simulink subsystem "DronePlantSubsystem"  (R2023b)
settings: Solver=VariableStepAuto  StartTime=0.0  StopTime=10.0  RelTol=1e-3
values from neighbouring files (symbols this model uses):
  Ax = 0.0    (= 0)    [drone_input_params.m]
  Ay = 0.0    (= 0)    [drone_input_params.m]
  Az = 0.0    (= 0)    [drone_input_params.m]
  b = 192.3208*10^(-7)    (= 1.923208e-05)    [drone_input_params.m]
  d = 4.003*10^(-7)    (= 4.003e-07)    [drone_input_params.m]
  g = 9.81    [drone_input_params.m]
  Ixx = 15.67*10^(-3)    (= 0.01567)    [drone_input_params.m]
  Iyy = 15.67*10^(-3)    (= 0.01567)    [drone_input_params.m]
  Izz = 28.346*10^(-3)    (= 0.028346)    [drone_input_params.m]
  Jr = 6.01*10^(-5)    (= 6.01e-05)    [drone_input_params.m]
  l = 0.3    [drone_input_params.m]
  m = weight/g    (= 0.815494393476)    [drone_input_params.m]
settings Model: Creator=FRESH  LastModifiedBy=FRESH

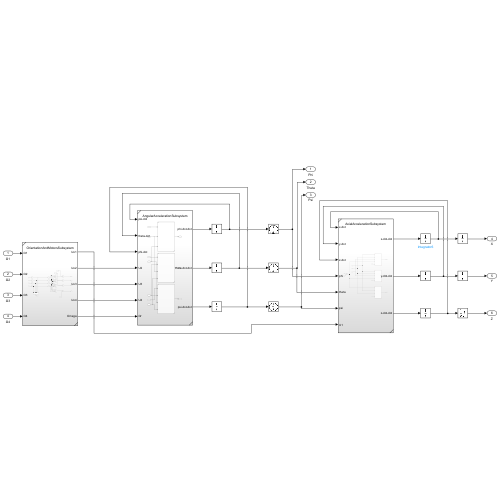
[thumbnail: Simulink's stored preview of the top-level diagram]
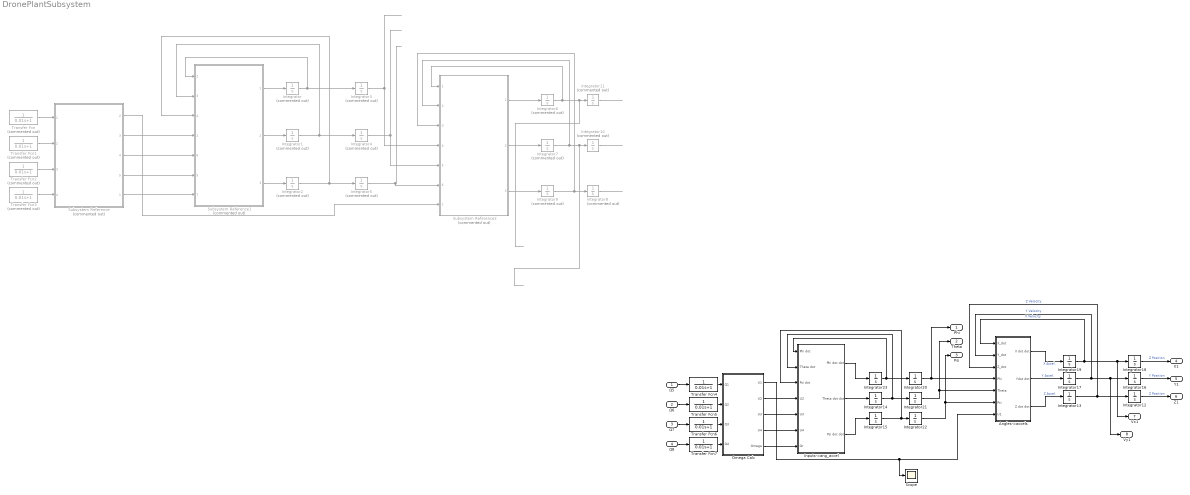
== system DronePlantSubsystem ==
  Ω5 : Inport
  Ω6 : Inport  Port=2
  Ω7 : Inport  Port=3
  Ω8 : Inport  Port=4
  Angles->accels : Subsystem
  Inputs->ang_accel : Subsystem
  Integrator{,1..2,6..7,9..11} (8 alike) : Integrator  Commented=on
  Integrator12 : Integrator  LimitOutput=on  LowerSaturationLimit=0
  Integrator{13,16..19,22..23} (7 alike) : Integrator
  Integrator14 : Integrator  UpperSaturationLimit=10000  LowerSaturationLimit=-10000
  Integrator15 : Integrator  UpperSaturationLimit=10000  LowerSaturationLimit=-10000
  Integrator20 : Integrator  WrapState=on  WrappedStateUpperValue=pi/2  WrappedStateLowerValue=-pi/2
  Integrator21 : Integrator  WrapState=on  WrappedStateUpperValue=pi/3  WrappedStateLowerValue=-pi/3
  Integrator3 : Integrator  Commented=on  WrapState=on
  Integrator4 : Integrator  Commented=on  WrapState=on
  Integrator5 : Integrator  Commented=on  WrapState=on
  Integrator8 : Integrator  Commented=on  LimitOutput=on  UpperSaturationLimit=0
  Omega Calc : Subsystem
  Scope : Scope
  Subsystem Reference : Subsystem  Commented=on  ReferencedSubsystem=OrientationAndMotorsSubsystem
      settings: PortSchema="{\"entries\":[{\"content\":{\"sides\":[{\"content\":{\"connectorIds\":[\"In1\",\"In2\",\"In3\",\"In4\"]},\"type\":\"ConnectorPlacement.EquallySpacedRectSide\",\"uuid\":\"54093c14-6905-4315-89a2-d57263587d77\"},{\"content\":{\"connectorIds\":[\"Out2\",\"Out3\",\"Out4\",\"Out5\",\"Out1\"],\"side\":\"RIGHT\"},\"type\":\"ConnectorPlacement.EquallySpacedRectSide\",\"uuid\":\"792b5cf1-0f94-4e71-8b93-1e59081231d9\"},{\"content\":{\"side\":\"TOP\"},\"type\":\"ConnectorPlacement.EquallySpacedRectSide\",\"uuid\":\"8a70e999-dff0-4dcb-8d8e-633240736e28\"}]},\"type\":\"ConnectorPlacement.EquallySpacedConnector\",\"uuid\":\"4c2f7de4-146f-41b0-aabc-cf54c6108d54\"}],\"packageUris\":[\"http://schema.mathworks.com/mf0/Connector/R2020b\"],\"version\":\"1.0\"}"
  Subsystem Reference1 : Subsystem  Commented=on  ReferencedSubsystem=AngularAccelerationSubsystem
      settings: PortSchema="{\"entries\":[{\"content\":{\"sides\":[{\"content\":{\"connectorIds\":[\"In2\",\"In3\",\"In4\",\"In1\",\"In6\",\"In5\",\"In7\"]},\"type\":\"ConnectorPlacement.EquallySpacedRectSide\",\"uuid\":\"e7cd80e4-513a-49bb-8a32-93ee463d1d18\"},{\"content\":{\"connectorIds\":[\"Out1\",\"Out2\",\"Out3\"],\"side\":\"RIGHT\"},\"type\":\"ConnectorPlacement.EquallySpacedRectSide\",\"uuid\":\"416d32a0-b191-4ff2-830a-04dcaeaab673\"},{\"content\":{\"side\":\"TOP\"},\"type\":\"ConnectorPlacement.EquallySpacedRectSide\",\"uuid\":\"e39a2d85-751d-4d15-b0f4-13a7a5828542\"}]},\"type\":\"ConnectorPlacement.EquallySpacedConnector\",\"uuid\":\"cd683958-b96b-4e10-be5c-088f75616717\"}],\"packageUris\":[\"http://schema.mathworks.com/mf0/Connector/R2020b\"],\"version\":\"1.0\"}"
  Subsystem Reference2 : Subsystem  Commented=on  ReferencedSubsystem=AxialAccelerationSubsystem
  Transfer Fcn{,1..3} (4 alike) : TransferFcn  Commented=on  Denominator=[0.01 1]
  Transfer Fcn{4..7} (4 alike) : TransferFcn  Denominator=[0.01 1]
  Phi : Outport  VectorParamsAs1DForOutWhenUnconnected=off
  Theta : Outport  Port=2  VectorParamsAs1DForOutWhenUnconnected=off
  Psi : Outport  Port=3  VectorParamsAs1DForOutWhenUnconnected=off
  X1 : Outport  Port=4  VectorParamsAs1DForOutWhenUnconnected=off
  Y1 : Outport  Port=5  VectorParamsAs1DForOutWhenUnconnected=off
  Z1 : Outport  Port=6  VectorParamsAs1DForOutWhenUnconnected=off
  Vx1 : Outport  Port=7  VectorParamsAs1DForOutWhenUnconnected=off
  Vy1 : Outport  Port=8  VectorParamsAs1DForOutWhenUnconnected=off
  wires:
  ? -> Transfer Fcn/1
  ? -> Transfer Fcn1/1
  ? -> Transfer Fcn2/1
  ? -> Transfer Fcn3/1
  Subsystem Reference/1 -> Subsystem Reference1/7
  Subsystem Reference/5 -> Subsystem Reference1/5
  Subsystem Reference/4 -> Subsystem Reference1/6
  Subsystem Reference/3 -> Subsystem Reference1/1
  Subsystem Reference1/1 -> Integrator/1
  Subsystem Reference1/2 -> Integrator1/1
  Subsystem Reference1/3 -> Integrator2/1
  Integrator/1 -> Integrator3/1, Subsystem Reference1/2
  Integrator1/1 -> Subsystem Reference1/3, Integrator4/1
  Integrator2/1 -> Subsystem Reference1/4, Integrator5/1
  Integrator5/1 -> Subsystem Reference2/6
  Integrator4/1 -> Subsystem Reference2/5
  Integrator3/1 -> Subsystem Reference2/4
  Subsystem Reference/2 -> Subsystem Reference2/7
  Subsystem Reference2/1 -> Integrator6/1
  Subsystem Reference2/2 -> Integrator7/1
  Subsystem Reference2/3 -> Integrator9/1
  Integrator7/1 -> Subsystem Reference2/2, Integrator10/1
  Integrator9/1 -> Integrator8/1, Subsystem Reference2/3
  Integrator11/1 -> ?
  Integrator10/1 -> ?
  Integrator8/1 -> ?
  Integrator6/1 -> Integrator11/1, Subsystem Reference2/1
  Transfer Fcn/1 -> Subsystem Reference/1
  Transfer Fcn1/1 -> Subsystem Reference/2
  Transfer Fcn2/1 -> Subsystem Reference/3
  Transfer Fcn3/1 -> Subsystem Reference/4
  Omega Calc/4(U4) -> Inputs->ang_accel/6(U4)
  Angles->accels/1(X dot dot) -> Integrator19/1  "X Accel."
  Ω8/1 -> Transfer Fcn7/1
  Ω7/1 -> Transfer Fcn6/1
  Transfer Fcn4/1 -> Omega Calc/1(Ω1)
  Omega Calc/5(Omega) -> Inputs->ang_accel/7(Ωr)
  Integrator18/1 -> X1/1  "Z Position"
  Ω5/1 -> Transfer Fcn4/1
  Integrator15/1 -> Integrator22/1, Inputs->ang_accel/3(Psi dot)
  Ω6/1 -> Transfer Fcn5/1
  Transfer Fcn5/1 -> Omega Calc/2(Ω2)
  Integrator23/1 -> Integrator20/1, Inputs->ang_accel/1(Phi dot)
  Integrator19/1 -> Integrator18/1, Vx1/1, Angles->accels/1(X_dot)  "X Velocity"
  Integrator20/1 -> Phi/1, Angles->accels/4(Phi)
  Inputs->ang_accel/3(Psi dot dot) -> Integrator15/1
  Inputs->ang_accel/1(Phi dot dot) -> Integrator23/1
  Integrator12/1 -> Z1/1  "Z Position"
  Omega Calc/2(U2) -> Inputs->ang_accel/4(U2)
  Integrator14/1 -> Integrator21/1, Inputs->ang_accel/2(Theta dot)
  Angles->accels/3(Z dot dot) -> Integrator13/1  "Z Accel."
  Integrator16/1 -> Y1/1  "Y Position"
  Angles->accels/2(Ydot dot) -> Integrator17/1  "Y Accel."
  Omega Calc/1(U1) -> Angles->accels/7(U1), Scope/1
  Inputs->ang_accel/2(Theta dot dot) -> Integrator14/1
  Transfer Fcn7/1 -> Omega Calc/4(Ω4)
  Integrator17/1 -> Integrator16/1, Vy1/1, Angles->accels/2(Y_dot)  "Y Velocity"
  Integrator13/1 -> Integrator12/1, Angles->accels/3(Z_dot)  "Z Velocity"
  Integrator22/1 -> Psi/1, Angles->accels/6(Psi)
  Transfer Fcn6/1 -> Omega Calc/3(Ω3)
  Integrator21/1 -> Theta/1, Angles->accels/5(Theta)
  Omega Calc/3(U3) -> Inputs->ang_accel/5(U3)

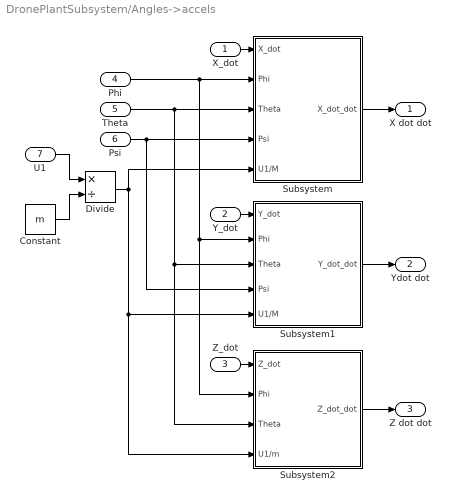
== system DronePlantSubsystem/Angles->accels ==
  X_dot : Inport
  Y_dot : Inport  Port=2
  Z_dot : Inport  Port=3
  Phi : Inport  Port=4
  Theta : Inport  Port=5
  Psi : Inport  Port=6
  U1 : Inport  Port=7
  Constant : Constant  Value=m
  Divide : Product  Inputs=*/
  Subsystem : Subsystem
  Subsystem1 : Subsystem
  Subsystem2 : Subsystem
  X dot dot : Outport  VectorParamsAs1DForOutWhenUnconnected=off
  Ydot dot : Outport  Port=2  VectorParamsAs1DForOutWhenUnconnected=off
  Z dot dot : Outport  Port=3  VectorParamsAs1DForOutWhenUnconnected=off
  wires:
  Z_dot/1 -> Subsystem2/1(Z_dot)
  Y_dot/1 -> Subsystem1/1(Y_dot)
  X_dot/1 -> Subsystem/1(X_dot)
  Psi/1 -> Subsystem/4(Psi), Subsystem1/4(Psi)
  Theta/1 -> Subsystem/3(Theta), Subsystem1/3(Theta), Subsystem2/3(Theta)
  Subsystem2/1(Z_dot_dot) -> Z dot dot/1
  Subsystem1/1(Y_dot_dot) -> Ydot dot/1
  Subsystem/1(X_dot_dot) -> X dot dot/1
  Divide/1 -> Subsystem1/5(U1/M), Subsystem2/4(U1/m), Subsystem/5(U1/M)
  Constant/1 -> Divide/2
  U1/1 -> Divide/1
  Phi/1 -> Subsystem/2(Phi), Subsystem1/2(Phi), Subsystem2/2(Phi)

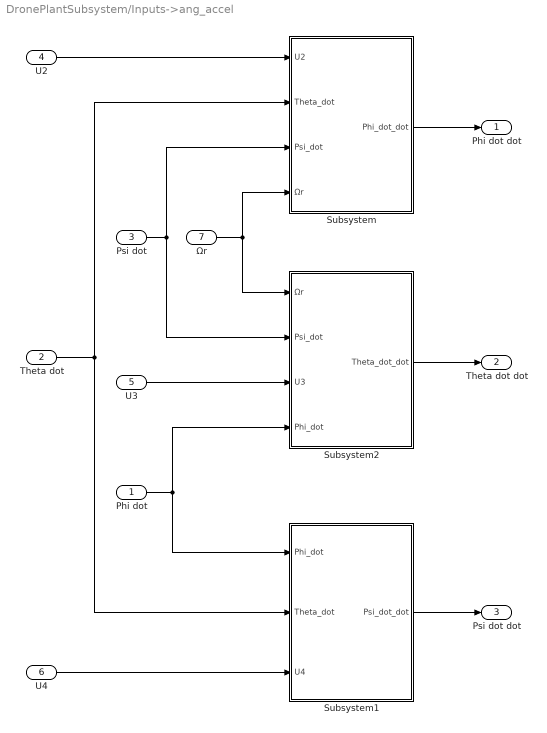
== system DronePlantSubsystem/Inputs->ang_accel ==
  Phi dot : Inport
  Theta dot : Inport  Port=2
  Psi dot : Inport  Port=3
  U2 : Inport  Port=4
  U3 : Inport  Port=5
  U4 : Inport  Port=6
  Ωr : Inport  Port=7
  Subsystem : Subsystem
  Subsystem1 : Subsystem
  Subsystem2 : Subsystem
  Phi dot dot : Outport  VectorParamsAs1DForOutWhenUnconnected=off
  Theta dot dot : Outport  Port=2  VectorParamsAs1DForOutWhenUnconnected=off
  Psi dot dot : Outport  Port=3  VectorParamsAs1DForOutWhenUnconnected=off
  wires:
  Phi dot/1 -> Subsystem1/1(Phi_dot), Subsystem2/4(Phi_dot)
  Theta dot/1 -> Subsystem1/2(Theta_dot), Subsystem/2(Theta_dot)
  Subsystem1/1(Psi_dot_dot) -> Psi dot dot/1
  Subsystem2/1(Theta_dot_dot) -> Theta dot dot/1
  Psi dot/1 -> Subsystem/3(Psi_dot), Subsystem2/2(Psi_dot)
  Ωr/1 -> Subsystem2/1(Ωr), Subsystem/4(Ωr)
  U2/1 -> Subsystem/1(U2)
  Subsystem/1(Phi_dot_dot) -> Phi dot dot/1
  U4/1 -> Subsystem1/3(U4)
  U3/1 -> Subsystem2/3(U3)

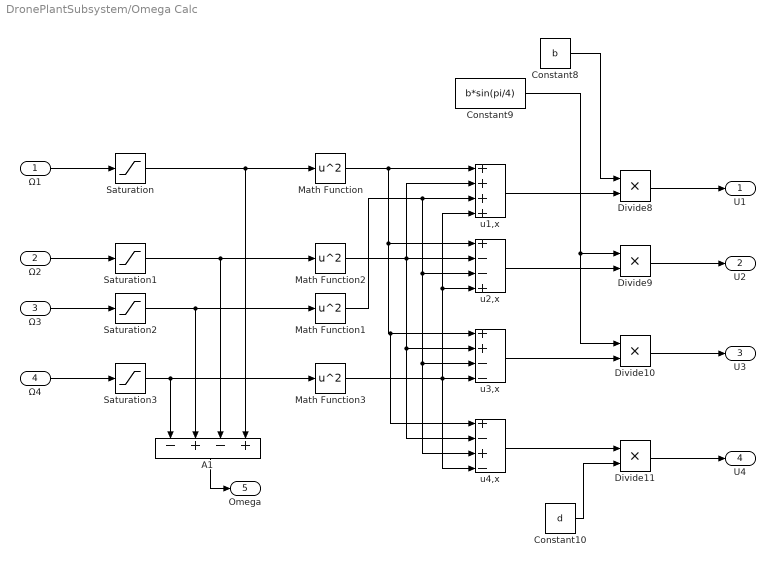
== system DronePlantSubsystem/Omega Calc ==
  Ω1 : Inport
  Ω2 : Inport  Port=2
  Ω3 : Inport  Port=3
  Ω4 : Inport  Port=4
  A1 : Sum  Inputs=-+-+
  Constant10 : Constant  Value=d
  Constant8 : Constant  Value=b
  Constant9 : Constant  Value=b*sin(pi/4)
  Divide{8..11} (4 alike) : Product  Inputs=**
  Math Function{,1..3} (4 alike) : Math  Operator=square  SignedPower=on
  Saturation{,1..3} (4 alike) : Saturate  UpperLimit=inf  LowerLimit=0
  u1,x : Sum  Inputs=++++
  u2,x : Sum  Inputs=+--+
  u3,x : Sum  Inputs=++--
  u4,x : Sum  Inputs=+-+-
  U1 : Outport  VectorParamsAs1DForOutWhenUnconnected=off
  U2 : Outport  Port=2  VectorParamsAs1DForOutWhenUnconnected=off
  U3 : Outport  Port=3  VectorParamsAs1DForOutWhenUnconnected=off
  U4 : Outport  Port=4  VectorParamsAs1DForOutWhenUnconnected=off
  Omega : Outport  Port=5  VectorParamsAs1DForOutWhenUnconnected=off
  wires:
  Saturation3/1 -> Math Function3/1, A1/1
  Saturation/1 -> A1/4, Math Function/1
  Saturation1/1 -> A1/3, Math Function2/1
  Saturation2/1 -> Math Function1/1, A1/2
  Ω4/1 -> Saturation3/1
  Ω3/1 -> Saturation2/1
  Ω2/1 -> Saturation1/1
  Ω1/1 -> Saturation/1
  Math Function3/1 -> u3,x/4, u4,x/4, u2,x/4, u1,x/4
  Math Function2/1 -> u2,x/2, u3,x/2, u4,x/2, u1,x/2
  Math Function1/1 -> u1,x/3, u2,x/3, u3,x/3, u4,x/3
  Math Function/1 -> u1,x/1, u2,x/1, u3,x/1, u4,x/1
  Divide11/1 -> U4/1
  Divide10/1 -> U3/1
  Divide9/1 -> U2/1
  Divide8/1 -> U1/1
  A1/1 -> Omega/1
  Constant8/1 -> Divide8/1
  u1,x/1 -> Divide8/2
  Constant9/1 -> Divide9/1, Divide10/1
  u2,x/1 -> Divide9/2
  u3,x/1 -> Divide10/2
  u4,x/1 -> Divide11/1
  Constant10/1 -> Divide11/2

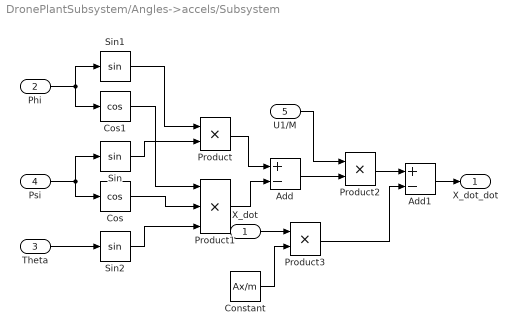
== system DronePlantSubsystem/Angles->accels/Subsystem ==
  X_dot : Inport
  Phi : Inport  Port=2
  Theta : Inport  Port=3
  Psi : Inport  Port=4
  U1/M : Inport  Port=5
  Add : Sum  Inputs=+-
  Add1 : Sum  Inputs=+-
  Constant : Constant  Value=Ax/m
  Cos : Trigonometry  Operator=cos
  Cos1 : Trigonometry  Operator=cos
  Product : Product
  Product1 : Product  Inputs=3
  Product2 : Product
  Product3 : Product
  Sin : Trigonometry
  Sin1 : Trigonometry
  Sin2 : Trigonometry
  X_dot_dot : Outport  VectorParamsAs1DForOutWhenUnconnected=off
  wires:
  Product3/1 -> Add1/2
  Constant/1 -> Product3/2
  X_dot/1 -> Product3/1
  Add1/1 -> X_dot_dot/1
  Product2/1 -> Add1/1
  Sin/1 -> Product/2
  Sin1/1 -> Product/1
  Sin2/1 -> Product1/3
  Cos/1 -> Product1/2
  Cos1/1 -> Product1/1
  Theta/1 -> Sin2/1
  Phi/1 -> Sin1/1, Cos1/1
  Psi/1 -> Sin/1, Cos/1
  Add/1 -> Product2/2
  U1/M/1 -> Product2/1
  Product/1 -> Add/1
  Product1/1 -> Add/2

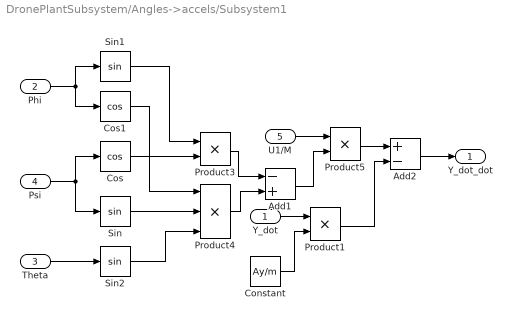
== system DronePlantSubsystem/Angles->accels/Subsystem1 ==
  Y_dot : Inport
  Phi : Inport  Port=2
  Theta : Inport  Port=3
  Psi : Inport  Port=4
  U1/M : Inport  Port=5
  Add1 : Sum  Inputs=-+
  Add2 : Sum  Inputs=+-
  Constant : Constant  Value=Ay/m
  Cos : Trigonometry  Operator=cos
  Cos1 : Trigonometry  Operator=cos
  Product1 : Product
  Product3 : Product
  Product4 : Product  Inputs=3
  Product5 : Product
  Sin : Trigonometry
  Sin1 : Trigonometry
  Sin2 : Trigonometry
  Y_dot_dot : Outport  VectorParamsAs1DForOutWhenUnconnected=off
  wires:
  Add2/1 -> Y_dot_dot/1
  Product5/1 -> Add2/1
  Product1/1 -> Add2/2
  Constant/1 -> Product1/2
  Y_dot/1 -> Product1/1
  Cos/1 -> Product3/2
  Sin1/1 -> Product3/1
  Sin2/1 -> Product4/3
  Sin/1 -> Product4/2
  Cos1/1 -> Product4/1
  Product3/1 -> Add1/1
  U1/M/1 -> Product5/1
  Product4/1 -> Add1/2
  Add1/1 -> Product5/2
  Theta/1 -> Sin2/1
  Phi/1 -> Sin1/1, Cos1/1
  Psi/1 -> Cos/1, Sin/1

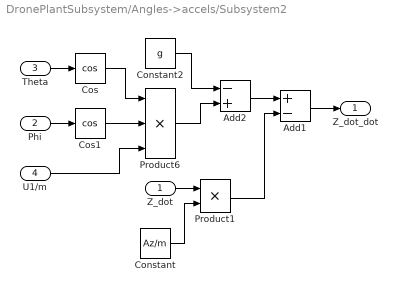
== system DronePlantSubsystem/Angles->accels/Subsystem2 ==
  Z_dot : Inport
  Phi : Inport  Port=2
  Theta : Inport  Port=3
  U1/m : Inport  Port=4
  Add1 : Sum  Inputs=+-
  Add2 : Sum  Inputs=-+
  Constant : Constant  Value=Az/m
  Constant2 : Constant  Value=g
  Cos : Trigonometry  Operator=cos
  Cos1 : Trigonometry  Operator=cos
  Product1 : Product
  Product6 : Product  Inputs=3
  Z_dot_dot : Outport  VectorParamsAs1DForOutWhenUnconnected=off
  wires:
  Add1/1 -> Z_dot_dot/1
  Add2/1 -> Add1/1
  Constant/1 -> Product1/2
  Z_dot/1 -> Product1/1
  Product1/1 -> Add1/2
  Cos1/1 -> Product6/2
  Product6/1 -> Add2/2
  Cos/1 -> Product6/1
  Constant2/1 -> Add2/1
  U1/m/1 -> Product6/3
  Theta/1 -> Cos/1
  Phi/1 -> Cos1/1

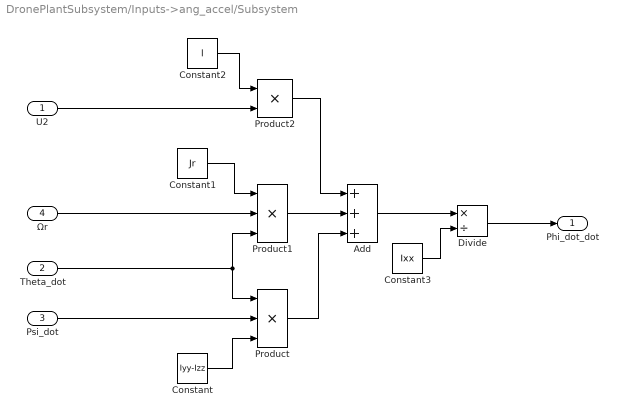
== system DronePlantSubsystem/Inputs->ang_accel/Subsystem ==
  U2 : Inport
  Theta_dot : Inport  Port=2
  Psi_dot : Inport  Port=3
  Ωr : Inport  Port=4
  Add : Sum  Inputs=+++
  Constant : Constant  Value=Iyy-Izz
  Constant1 : Constant  Value=Jr
  Constant2 : Constant  Value=l
  Constant3 : Constant  Value=Ixx
  Divide : Product  Inputs=*/
  Product : Product  Inputs=3
  Product1 : Product  Inputs=3
  Product2 : Product
  Phi_dot_dot : Outport  VectorParamsAs1DForOutWhenUnconnected=off
  wires:
  Divide/1 -> Phi_dot_dot/1
  Constant3/1 -> Divide/2
  Add/1 -> Divide/1
  Product/1 -> Add/3
  Product2/1 -> Add/1
  Product1/1 -> Add/2
  Constant2/1 -> Product2/1
  U2/1 -> Product2/2
  Constant1/1 -> Product1/1
  Ωr/1 -> Product1/2
  Constant/1 -> Product/3
  Theta_dot/1 -> Product1/3, Product/1
  Psi_dot/1 -> Product/2

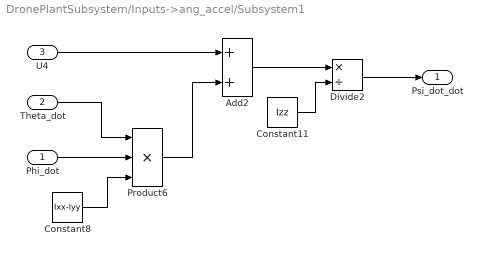
== system DronePlantSubsystem/Inputs->ang_accel/Subsystem1 ==
  Phi_dot : Inport
  Theta_dot : Inport  Port=2
  U4 : Inport  Port=3
  Add2 : Sum
  Constant11 : Constant  Value=Izz
  Constant8 : Constant  Value=Ixx-Iyy
  Divide2 : Product  Inputs=*/
  Product6 : Product  Inputs=3
  Psi_dot_dot : Outport  VectorParamsAs1DForOutWhenUnconnected=off
  wires:
  U4/1 -> Add2/1
  Product6/1 -> Add2/2
  Divide2/1 -> Psi_dot_dot/1
  Constant11/1 -> Divide2/2
  Add2/1 -> Divide2/1
  Constant8/1 -> Product6/3
  Phi_dot/1 -> Product6/2
  Theta_dot/1 -> Product6/1

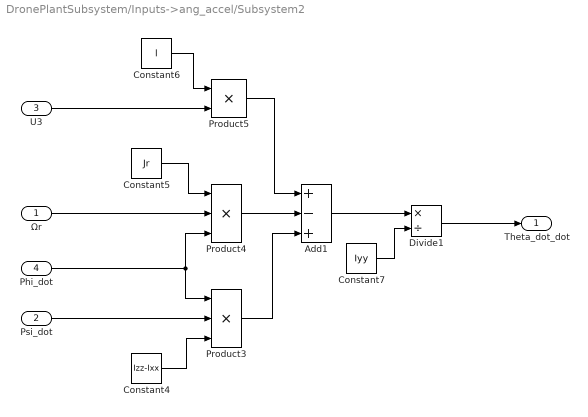
== system DronePlantSubsystem/Inputs->ang_accel/Subsystem2 ==
  Ωr : Inport
  Psi_dot : Inport  Port=2
  U3 : Inport  Port=3
  Phi_dot : Inport  Port=4
  Add1 : Sum  Inputs=+-+
  Constant4 : Constant  Value=Izz-Ixx
  Constant5 : Constant  Value=Jr
  Constant6 : Constant  Value=l
  Constant7 : Constant  Value=Iyy
  Divide1 : Product  Inputs=*/
  Product3 : Product  Inputs=3
  Product4 : Product  Inputs=3
  Product5 : Product
  Theta_dot_dot : Outport  VectorParamsAs1DForOutWhenUnconnected=off
  wires:
  Divide1/1 -> Theta_dot_dot/1
  Constant7/1 -> Divide1/2
  Add1/1 -> Divide1/1
  Product3/1 -> Add1/3
  Product5/1 -> Add1/1
  Product4/1 -> Add1/2
  Constant6/1 -> Product5/1
  U3/1 -> Product5/2
  Constant5/1 -> Product4/1
  Constant4/1 -> Product3/3
  Ωr/1 -> Product4/2
  Phi_dot/1 -> Product4/3, Product3/1
  Psi_dot/1 -> Product3/2
